simulink model "simulate_copter"  (R2026a)
settings: Solver=VariableStepAuto  StopTime=20
undefined symbols (not defined in the file or in its folder): P
settings Model: Creator=Kiril  LastModifiedBy=Kiril

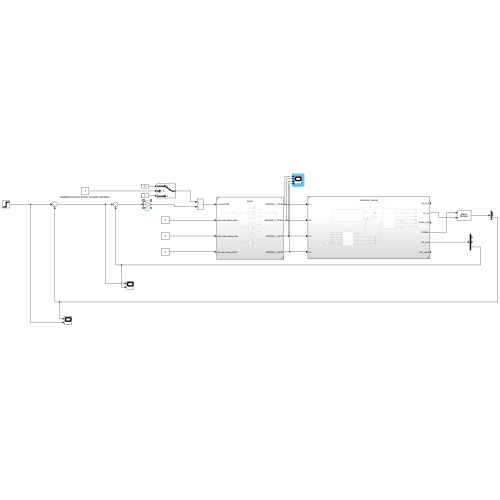
[thumbnail: Simulink's stored preview of the top-level diagram]
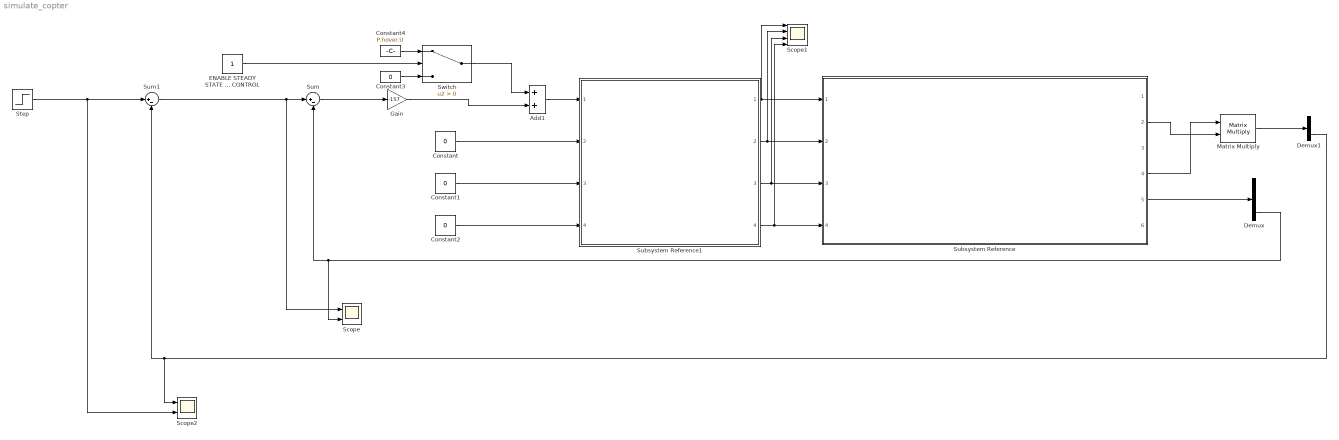
== system simulate_copter ==
  Add1 : Sum
  Constant{,1..3} (4 alike) : Constant  Value=0
  Constant4 : Constant  Value=P.hover.U
  Demux : Demux  Outputs=3
  Demux1 : Demux  Outputs=3
  ENABLE STEADY STATE HOVER CONTROL : Constant
  Gain : Gain  Gain=-157
  Matrix Multiply : Product  Multiplication=Matrix(*)
  Scope : Scope  NumInputPorts=2
      settings: ActiveDisplayYMinimum=-1.0627421021082206  ActiveDisplayYMaximum=2.0867248032657875
  Scope1 : Scope  NumInputPorts=4
      settings: ActiveDisplayYMinimum=72.881589615881126  ActiveDisplayYMaximum=138.51885888789394
  Scope2 : Scope  NumInputPorts=2
      settings: ActiveDisplayYMinimum=0.24240965238986989  ActiveDisplayYMaximum=1.4540822435150336  DataLoggingVariableName=ScopeData11
  Step : Step  SampleTime=0
  Subsystem Reference : Subsystem  ReferencedSubsystem=nonlinear_model
  Subsystem Reference1 : Subsystem  ReferencedSubsystem=mixer
  Sum : Sum  Inputs=|+-
  Sum1 : Sum  Inputs=|+-
  Switch : Switch  Criteria=u2 > Threshold  SaturateOnIntegerOverflow=off  InputSameDT=off
  wires:
  Subsystem Reference1/1 -> Scope1/1, Subsystem Reference/1
  Subsystem Reference1/2 -> Subsystem Reference/2, Scope1/2
  Subsystem Reference1/3 -> Scope1/3, Subsystem Reference/3
  Subsystem Reference1/4 -> Scope1/4, Subsystem Reference/4
  Subsystem Reference/5 -> Demux/1
  Demux/3 -> Scope/2, Sum/2
  Sum/1 -> Gain/1
  Constant/1 -> Subsystem Reference1/2
  Constant1/1 -> Subsystem Reference1/3
  Constant2/1 -> Subsystem Reference1/4
  Subsystem Reference/4 -> Matrix Multiply/1
  Subsystem Reference/2 -> Matrix Multiply/2
  Matrix Multiply/1 -> Demux1/1
  Step/1 -> Scope2/2, Sum1/1
  Demux1/3 -> Scope2/1, Sum1/2
  Sum1/1 -> Sum/1, Scope/1
  Switch/1 -> Add1/1
  Constant3/1 -> Switch/3
  Constant4/1 -> Switch/1
  ENABLE STEADY STATE HOVER CONTROL/1 -> Switch/2
  Add1/1 -> Subsystem Reference1/1
  Gain/1 -> Add1/2
